simulink model "exp3_2_elastic_joint_estimation"  (R2020b)
settings: Solver=FixedStepDiscrete  StartTime=0.0  StopTime=10  FixedStep=Ts  RelTol=1e-3
undefined symbols (not defined in the file): DiscIntNeverNeededParam, National_Instruments, PCI, sens, Ts
libraries: sldrtlib x4, simulink x2
settings Model: ExtModeTrigDuration=100000  Creator=umbe  LastModifiedBy=irong
settings RTWCC: Description=Simulink Desktop Real-Time  SystemTargetFile=sldrt.tlc  TemplateMakefile=sldrt.tmf  RTWCompilerOptimization=on
settings CodeAppCC: MaxIdLength=95
settings SimulinkDesktopRealTimeCC: TargetPreCompLibLocation=D:\MATLAB\R2020b\toolbox\sldrt\lib\win64

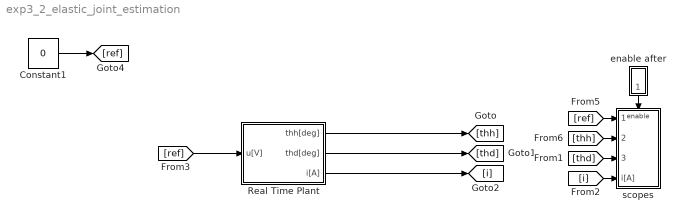
== system exp3_2_elastic_joint_estimation ==
  Constant1 : Constant  Value=0
  Real Time Plant : Subsystem
  enable after : Subsystem
  scopes : Subsystem
  wires:
  [ref] -> Real Time Plant/1(u[V])
  Real Time Plant/1(thh[deg]) -> [thh]
  Real Time Plant/2(thd[deg]) -> [thd]
  Real Time Plant/3(i[A]) -> [i]
  Constant1/1 -> [ref]
  [ref] -> scopes/1(ref[deg])
  [thh] -> scopes/2(thh[deg])
  [thd] -> scopes/3(thd[deg])
  [i] -> scopes/4(i[A])
  enable after/1(1.0 s) -> scopes/Enable

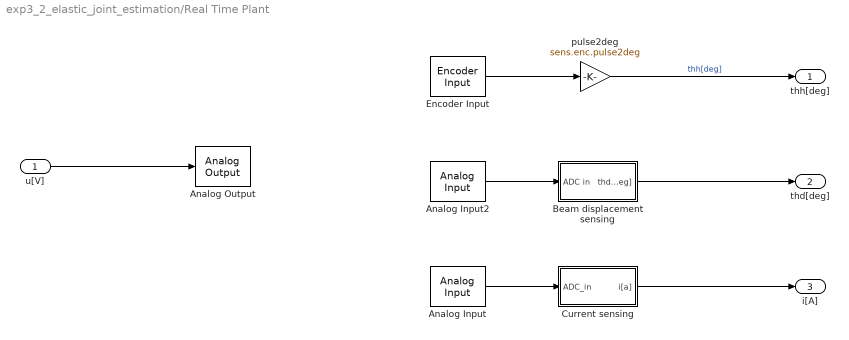
== system exp3_2_elastic_joint_estimation/Real Time Plant ==
  u[V] : Inport
  Analog Input : sldrtlib/Analog Input  SampleTime=Ts  MaxMissedTicks=10  ShowMissedTicks=off  YieldWhenWaiting=off  DrvName=National_Instruments/PCI-6221  DrvAddress=4294967295  DrvOptions=[0 0 0 2 0]  Channels=[1 2]  RangeMode=1  VoltRange=1  DataType=1
      settings: AttributesFormatString=National Instruments\nPCI-6221 [auto]
  Analog Input2 : sldrtlib/Analog Input  SampleTime=Ts  MaxMissedTicks=10  ShowMissedTicks=off  YieldWhenWaiting=off  DrvName=National_Instruments/PCI-6221  DrvAddress=4294967295  DrvOptions=[0 0 0 2 0]  Channels=[3,4]  RangeMode=1  VoltRange=2  DataType=1
      settings: AttributesFormatString=National Instruments\nPCI-6221 [auto]
  Analog Output : sldrtlib/Analog Output  SampleTime=Ts  MaxMissedTicks=10  ShowMissedTicks=off  YieldWhenWaiting=off  DrvName=National_Instruments/PCI-6221  DrvAddress=4294967295  DrvOptions=[0 0 0 2 0]  Channels=1  RangeMode=1  VoltRange=1  InitialValue=0  FinalValue=0
      settings: AttributesFormatString=National Instruments\nPCI-6221 [auto]
  Beam displacement sensing : Subsystem
  Current sensing : Subsystem
  Encoder Input : sldrtlib/Encoder Input  SampleTime=Ts  MaxMissedTicks=10  ShowMissedTicks=off  YieldWhenWaiting=off  DrvName=National_Instruments/PCI-6221  DrvAddress=4294967295  DrvOptions=[0 0 0 2 0]  Channels=1  QuadMode=3  IndexPulse=1  InputFilter=Inf  DataType=1
      settings: AttributesFormatString=National Instruments\nPCI-6221 [auto]
  pulse2deg : Gain  Gain=sens.enc.pulse2deg
  thh[deg] : Outport
  thd[deg] : Outport  Port=2
  i[A] : Outport  Port=3
  wires:
  pulse2deg/1 -> thh[deg]/1  "thh[deg]"
  Beam displacement sensing/1(thd[deg]) -> thd[deg]/1
  Analog Input/1 -> Current sensing/1(ADC_in)
  Analog Input2/1 -> Beam displacement sensing/1(ADC in)
  u[V]/1 -> Analog Output/1
  Encoder Input/1 -> pulse2deg/1
  Current sensing/1(i[a]) -> i[A]/1

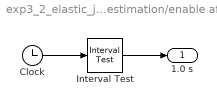
== system exp3_2_elastic_joint_estimation/enable after ==
  Clock : Clock
  Interval Test : simulink/Logic and Bit Operations/Interval Test  IntervalClosedRight=on  uplimit=inf  IntervalClosedLeft=on  lowlimit=1  OutDataTypeStr=boolean
  1.0 s : Outport
  wires:
  Clock/1 -> Interval Test/1
  Interval Test/1 -> 1.0 s/1

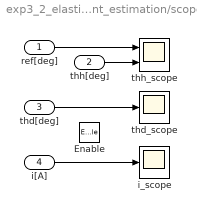
== system exp3_2_elastic_joint_estimation/scopes ==
  ref[deg] : Inport
  thh[deg] : Inport  Port=2
  thd[deg] : Inport  Port=3
  i[A] : Inport  Port=4
  Enable : EnablePort
  i_scope : Scope
  thd_scope : Scope
  thh_scope : Scope  NumInputPorts=2
  wires:
  ref[deg]/1 -> thh_scope/1
  thh[deg]/1 -> thh_scope/2
  i[A]/1 -> i_scope/1
  thd[deg]/1 -> thd_scope/1

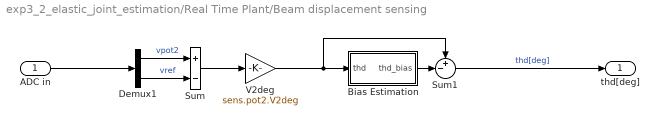
== system exp3_2_elastic_joint_estimation/Real Time Plant/Beam displacement sensing ==
  ADC in : Inport
  Bias Estimation : Subsystem
  Demux1 : Demux  Outputs=2
  Sum : Sum  Inputs=+-
  Sum1 : Sum  Inputs=+-|
  V2deg : Gain  Gain=sens.pot2.V2deg
  thd[deg] : Outport
  wires:
  ADC in/1 -> Demux1/1
  V2deg/1 -> Bias Estimation/1(thd), Sum1/1
  Sum1/1 -> thd[deg]/1  "thd[deg]"
  Demux1/2 -> Sum/2  "vref"
  Demux1/1 -> Sum/1  "vpot2"
  Sum/1 -> V2deg/1
  Bias Estimation/1(thd_bias) -> Sum1/2

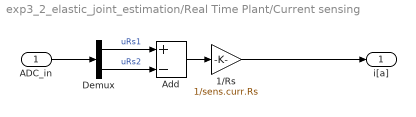
== system exp3_2_elastic_joint_estimation/Real Time Plant/Current sensing ==
  ADC_in : Inport
  1/Rs : Gain  Gain=1/sens.curr.Rs
  Add : Sum  Inputs=+-
  Demux : Demux  Outputs=2
  i[a] : Outport
  wires:
  Demux/1 -> Add/1  "uRs1"
  Demux/2 -> Add/2  "uRs2"
  Add/1 -> 1/Rs/1
  ADC_in/1 -> Demux/1
  1/Rs/1 -> i[a]/1

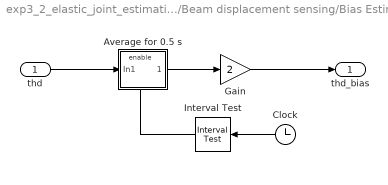
== system exp3_2_elastic_joint_estimation/Real Time Plant/Beam displacement sensing/Bias Estimation ==
  thd : Inport
  Average for 0.5 s : Subsystem
  Clock : Clock
  Gain : Gain  Gain=2
  Interval Test : simulink/Logic and Bit Operations/Interval Test  IntervalClosedRight=on  uplimit=0.7  IntervalClosedLeft=on  lowlimit=0.2  OutDataTypeStr=boolean
  thd_bias : Outport
  wires:
  Gain/1 -> thd_bias/1
  Average for 0.5 s/1(Out1) -> Gain/1
  Clock/1 -> Interval Test/1
  thd/1 -> Average for 0.5 s/1(In1)
  Interval Test/1 -> Average for 0.5 s/Enable

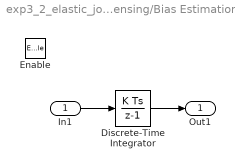
== system exp3_2_elastic_joint_estimation/Real Time Plant/Beam displacement sensing/Bias Estimation/Average for 0.5 s ==
  In1 : Inport
  Enable : EnablePort
  Discrete-Time Integrator : DiscreteIntegrator  SampleTime=Ts  ICPrevOutput=DiscIntNeverNeededParam  ICPrevScaledInput=DiscIntNeverNeededParam
  Out1 : Outport
  wires:
  Discrete-Time Integrator/1 -> Out1/1
  In1/1 -> Discrete-Time Integrator/1
